simulink model "part3_4"  (R2022a)
settings: Solver=VariableStepAuto  StartTime=0.0  StopTime=10.0  RelTol=1e-3
settings Model: Creator=HP  LastModifiedBy=HP

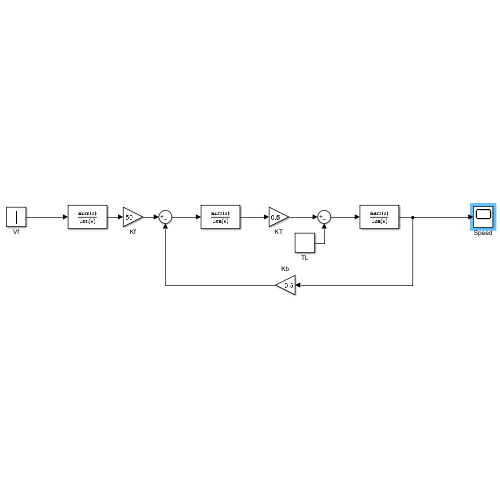
[thumbnail: Simulink's stored preview of the top-level diagram]
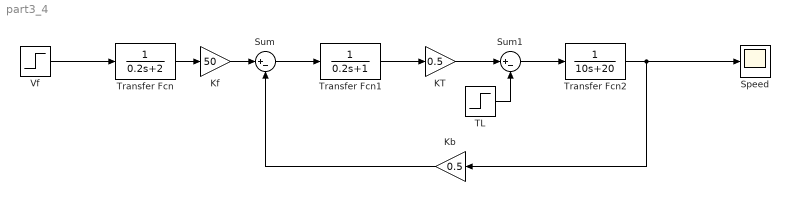
== system part3_4 ==
  KT : Gain  Gain=0.5
  Kb : Gain  Gain=0.5
  Kf : Gain  Gain=50
  Speed : Scope
  Sum : Sum  Inputs=|+-
  Sum1 : Sum  Inputs=|+-
  TL : Step  After=0  SampleTime=0
  Transfer Fcn : TransferFcn  Denominator=[0.2 2]
  Transfer Fcn1 : TransferFcn  Denominator=[0.2 1]
  Transfer Fcn2 : TransferFcn  Denominator=[10 20]
  Vf : Step  Time=0  SampleTime=0
  wires:
  Transfer Fcn/1 -> Kf/1
  Kf/1 -> Sum/1
  Sum/1 -> Transfer Fcn1/1
  KT/1 -> Sum1/1
  Transfer Fcn1/1 -> KT/1
  TL/1 -> Sum1/2
  Kb/1 -> Sum/2
  Sum1/1 -> Transfer Fcn2/1
  Transfer Fcn2/1 -> Speed/1, Kb/1
  Vf/1 -> Transfer Fcn/1
